simulink model "Cau_3_TDM_PAM"  (R2019a)
settings: Solver=VariableStepAuto  StartTime=0.0  StopTime=10.0  RelTol=1e-3
libraries: dsparch4 x2, dspsigops x2
settings Model: Creator=Thanh_Hai  LastModifiedBy=Thanh_Hai

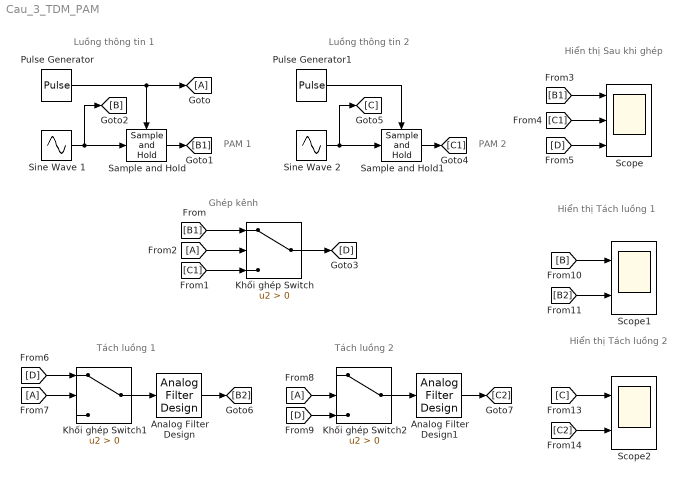
== system Cau_3_TDM_PAM ==
  note: Luồng thông tin 1
  note: PAM 1
  note: Luồng thông tin 2
  note: PAM 2
  note: Ghép kênh
  note: Hiển thị
      | Sau khi ghép
  note: Tách luồng 1
  note: Tách luồng 2
  note: Hiển thị
      | Tách luồng 1
  note: Hiển thị
      | Tách luồng 2
  "Analog Filter Design " : dsparch4/Analog Filter Design  method=Butterworth  filttype=Lowpass  N=12  Wlo=2*pi*2500  Whi=80  Rp=2  Rs=40
  Analog Filter Design1 : dsparch4/Analog Filter Design  method=Butterworth  filttype=Lowpass  N=12  Wlo=2*pi*1500  Whi=80  Rp=2  Rs=40
  Khối ghép Switch : Switch  Criteria=u2 > Threshold
  Khối ghép Switch1 : Switch  Criteria=u2 > Threshold
  Khối ghép Switch2 : Switch  Criteria=u2 > Threshold
  "Pulse Generator " : DiscretePulseGenerator  PulseType=Time based  Period=1/8000  PulseWidth=50
  Pulse Generator1 : DiscretePulseGenerator  PulseType=Time based  Period=1/8000  PulseWidth=50  PhaseDelay=1/16000
  "Sample and Hold " : dspsigops/Sample and Hold  trig=Rising edge  initCond=0  latchinput=off
  Sample and Hold1 : dspsigops/Sample and Hold  trig=Rising edge  initCond=0  latchinput=off
  Scope : Scope  NumInputPorts=3
  Scope1 : Scope  NumInputPorts=2
  Scope2 : Scope  NumInputPorts=2
  Sine Wave 1 : Sin  Frequency=2*pi*2000  SampleTime=1/64000
  Sine Wave 2 : Sin  Frequency=2*pi*1000  SampleTime=1/64000
  wires:
  Sine Wave 1/1 -> [B], "Sample and Hold "/1
  "Pulse Generator "/1 -> [A], "Sample and Hold "/Trigger
  "Sample and Hold "/1 -> [B1]
  Sample and Hold1/1 -> [C1]
  Sine Wave 2/1 -> [C], Sample and Hold1/1
  Pulse Generator1/1 -> Sample and Hold1/Trigger
  [B1] -> Khối ghép Switch/1
  [C1] -> Khối ghép Switch/3
  [A] -> Khối ghép Switch/2
  Khối ghép Switch/1 -> [D]
  [D] -> Scope/3
  [C1] -> Scope/2
  [B1] -> Scope/1
  Khối ghép Switch1/1 -> "Analog Filter Design "/1
  Khối ghép Switch2/1 -> Analog Filter Design1/1
  [D] -> Khối ghép Switch1/1
  [A] -> Khối ghép Switch1/2
  "Analog Filter Design "/1 -> [B2]
  [A] -> Khối ghép Switch2/2
  [D] -> Khối ghép Switch2/3
  Analog Filter Design1/1 -> [C2]
  [B2] -> Scope1/2
  [B] -> Scope1/1
  [C2] -> Scope2/2
  [C] -> Scope2/1
